simulink model "sistemaLineare3"  (R2025b)
settings: Solver=VariableStepAuto  StartTime=0.0  StopTime=10  RelTol=1e-3
values from neighbouring files (symbols this model uses):
  A_num = double(subs(A_eq, {J0, J1, J2, J3, J4, psi1, psi2, psi3, psi4, beta, k, theta_e}, {J0_val, J1_val, J2_val, J3_val, J4_val, psi1_val, psi2_val, psi3_val, psi4_val, beta_val, k_val, theta_e_val}))    [codiceProgetto3.m]
  B_num = double(subs(B_eq, {J0, J1, J2, J3, J4, psi1, psi2, psi3, psi4, beta, k, theta_e}, {J0_val, J1_val, J2_val, J3_val, J4_val, psi1_val, psi2_val, psi3_val, psi4_val, beta_val, k_val, theta_e_val}))    [codiceProgetto3.m]
  C_num = double(C_eq)    [codiceProgetto3.m]
  D_num = double(D_eq)    [codiceProgetto3.m]
libraries: cstblocks x1
settings Model: Creator=singh  LastModifiedBy=ospite

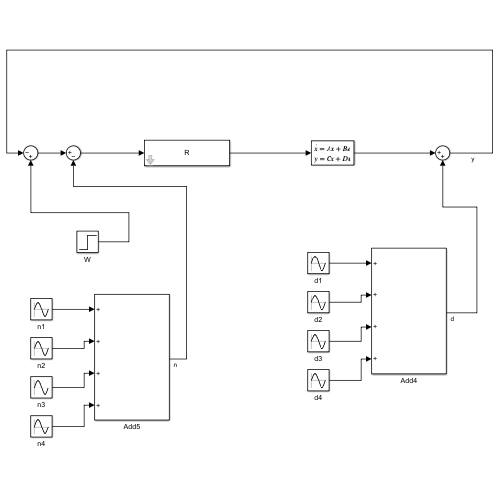
[thumbnail: Simulink's stored preview of the top-level diagram]
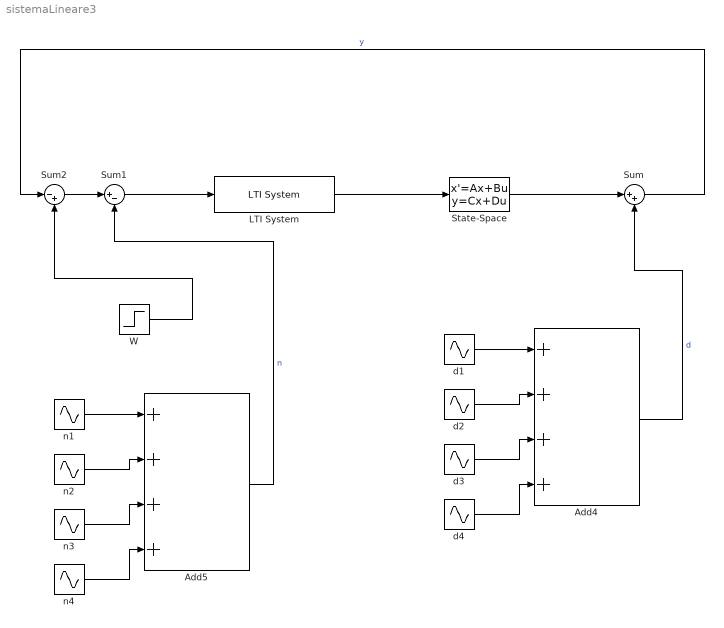
== system sistemaLineare3 ==
  Add4 : Sum  Inputs=++++
  Add5 : Sum  Inputs=++++
  LTI System : cstblocks/LTI System  sys=R  IC=[]  PadeOrder=0
  State-Space : StateSpace  A=A_num  B=B_num  C=C_num  D=D_num  InitialCondition=0
  Sum : Sum  Inputs=|++
  Sum1 : Sum  Inputs=|+-
  Sum2 : Sum  Inputs=|-+
  W : Step  Time=0  SampleTime=0
  d1 : Sin  Frequency=0.1*1  SampleTime=0
  d2 : Sin  Frequency=0.1*2  SampleTime=0
  d3 : Sin  Frequency=0.1*3  SampleTime=0
  d4 : Sin  Frequency=0.1*4  SampleTime=0
  n1 : Sin  Frequency=50000*1  SampleTime=0
  n2 : Sin  Frequency=50000*2  SampleTime=0
  n3 : Sin  Frequency=50000*3  SampleTime=0
  n4 : Sin  Frequency=50000*4  SampleTime=0
  wires:
  d2/1 -> Add4/2
  Sum2/1 -> Sum1/1
  d3/1 -> Add4/3
  n2/1 -> Add5/2
  Sum1/1 -> LTI System/1
  Add4/1 -> Sum/2  "d"
  n4/1 -> Add5/4
  Add5/1 -> Sum1/2  "n"
  LTI System/1 -> State-Space/1
  Sum/1 -> Sum2/1  "y"
  d4/1 -> Add4/4
  d1/1 -> Add4/1
  W/1 -> Sum2/2
  n1/1 -> Add5/1
  n3/1 -> Add5/3
  State-Space/1 -> Sum/1
